simulink model "SUB_CanDm1"  (R2018b)
settings: Solver=VariableStepDiscrete  StartTime=0.0  StopTime=10  RelTol=1e-3
PreLoadFcn:
  | if(exist('MBDS_ModelCallback', 'file'))
  |    MBDS_ModelCallback('PreLoad');
  | end
PostLoadFcn:
  | if(exist('MBDS_ModelCallback', 'file'))
  |    MBDS_ModelCallback('PostLoad');
  | end
InitFcn:
  | if(exist('MBDS_ModelCallback', 'file'))
  |    MBDS_ModelCallback('Init');
  | end
StartFcn:
  | if(exist('MBDS_ModelCallback', 'file'))
  |    MBDS_ModelCallback('Start');
  | end
StopFcn:
  | if(exist('MBDS_ModelCallback', 'file'))
  |    MBDS_ModelCallback('Stop');
  | end
undefined symbols (not defined in the file): sigbuilder_block
libraries: KIBES_Signal x47, simulink x1
(part 2 of 2)

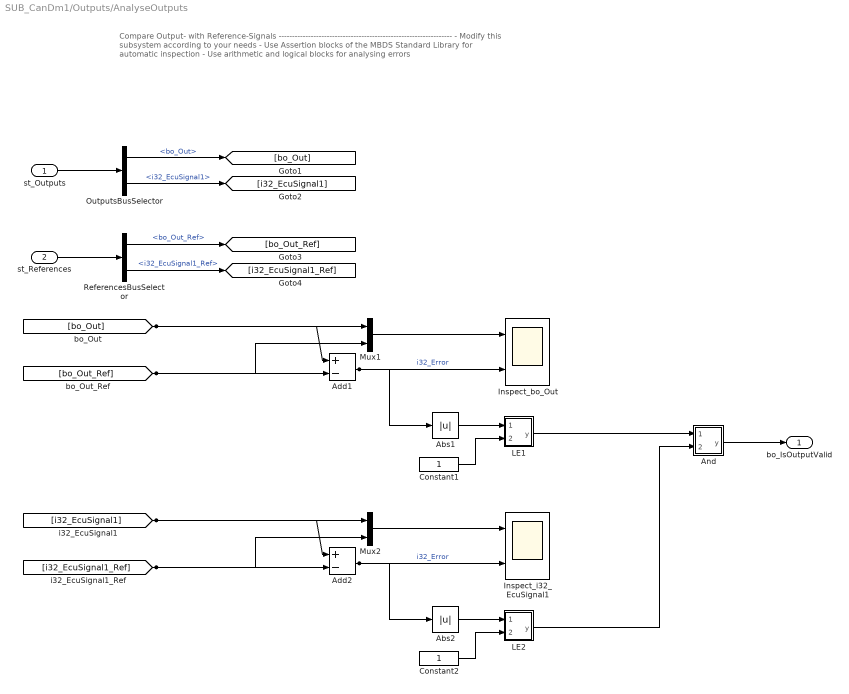
== system SUB_CanDm1/Outputs/AnalyseOutputs ==
  note: Compare Output- with Reference-Signals
      | -----------------------------------------------------------------
      | - Modify this subsystem according to your needs
      | -  Use Assertion blocks of the MBDS Standard Library for automatic inspection
      | - Use arithmetic and logical blocks for analysing errors
  st_Outputs : Inport  InitFcn=|
      | try
      |    MBDS_BlockCallback('Update', gcb);
      | end
  st_References : Inport  InitFcn=|  Port=2
      | try
      |    MBDS_BlockCallback('Update', gcb);
      | end
  Abs1 : Abs  InitFcn=|  OutDataTypeStr=Inherit: Inherit via back propagation
      | if(exist('MBDS_BlockCallback', 'file'))
      |    MBDS_BlockCallback('Update', gcb);  
      | end
      settings: AttributesFormatString=Saturate: %<SaturateOnIntegerOverflow>
  Abs2 : Abs  InitFcn=|  OutDataTypeStr=Inherit: Inherit via back propagation
      | if(exist('MBDS_BlockCallback', 'file'))
      |    MBDS_BlockCallback('Update', gcb);  
      | end
      settings: AttributesFormatString=Saturate: %<SaturateOnIntegerOverflow>
  Add1 : Sum  InitFcn=|  Inputs=+-  OutDataTypeStr=int32  SaturateOnIntegerOverflow=on  InputSameDT=on
      | if(exist('MBDS_BlockCallback', 'file'))
      |    MBDS_BlockCallback('Update', gcb);  
      | end
      settings: AttributesFormatString=Saturate: %<SaturateOnIntegerOverflow>
  Add2 : Sum  InitFcn=|  Inputs=+-  OutDataTypeStr=int32  SaturateOnIntegerOverflow=on  InputSameDT=on
      | if(exist('MBDS_BlockCallback', 'file'))
      |    MBDS_BlockCallback('Update', gcb);  
      | end
      settings: AttributesFormatString=Saturate: %<SaturateOnIntegerOverflow>
  And : Subsystem  InitFcn=|  mask(AND){MBDS_LibraryBlock=on, BitwiseMode=off, Inputs=2, UseBitMask=off, BitMask='A7', OutDataTypeStr=Inherit: Inherit via back propagation, MBDS_BlockVersion=08.20.02}
      | if(exist('MBDS_BlockCallback', 'file'))
      |    MBDS_BlockCallback('Update', gcb);
      | end
      mask prompts: MBDS_LibraryBlock "MBDS library block"; BitwiseMode "Use 'bitwise' mode"; Inputs "Number of input ports:"; UseBitMask "Use bit mask"; BitMask "Bit mask:"; OutDataTypeStr "Output data type:"; MBDS_BlockVersion "Version:"
      mask help: Logical or bitwise AND operator. For multiple inputs, operators are applied across the inputs. For a single input, operators are applied across the input vector. In bitwise mode a bit mask can be applied onto single input signals.
      mask init:
      | if(exist('MBDS_BlockCallback', 'file'))
      |    MBDS_BlockCallback('Init', gcb);
      | else
      |    % Disable all mask parameters
      |    MaskEnables = get_param(gcb, 'MaskEnables');
      |    for k = [1:length(MaskEnables)]
      |       MaskEnables{k} = 'off';
      |    end
      |    if(~isequal(MaskEnables, get_param(gcb, 'MaskEnables')))
      |       set_param(gcb, 'MaskEnables', MaskEnables);
      |    end
      | end
      mask Help: eval(['open([workdir(''library_dir:''),''\Blockset\help\'',get_param(gcb,''MaskType''),''.html''])'])
      mask Callback BitwiseMode:
      | if(exist('MBDS_BlockCallback', 'file'))
      |    MBDS_BlockCallback('BitwiseMode', gcb);
      | end
      mask Callback Inputs:
      | if(exist('MBDS_BlockCallback', 'file'))
      |    MBDS_BlockCallback('Inputs', gcb);
      | end
      mask Callback UseBitMask:
      | if(exist('MBDS_BlockCallback', 'file'))
      |    MBDS_BlockCallback('UseBitMask', gcb);
      | end
      mask Callback BitMask:
      | if(exist('MBDS_BlockCallback', 'file'))
      |    MBDS_BlockCallback('BitMask', gcb);
      | end
      mask TypeOptions OutDataTypeStr: Inherit: Inherit via back propagation | int8 | uint8 | int16 | uint16 | int32 | uint32 | boolean
      mask Callback OutDataTypeStr:
      | % Adopt Value
      | if(exist('MBDS_BlockCallback', 'file'))
      |    MBDS_BlockCallback('OutDataTypeStr', gcb);
      | end
      mask DialogControl ParameterTabVar0 Prompt: Main
      mask DialogControl ParameterTabVar01 Prompt: Signal Attributes
      mask DialogControl ParameterTabVar012 Prompt: Version
      mask Display:
      | % Show icon or block text
      | if(UseBitMask)
      |    if(isnumeric(BitMask))
      |       BitMaskString = ['0x',dec2hex(floor(BitMask))];
      |    elseif(ischar(BitMask))
      |       BitMaskString = ['0x',upper(BitMask)];
      |    else
      |       BitMaskString = '???';
      |    end
      |    disp(sprintf(['AND\n', BitMaskString]))
      | else
      |    disp('AND')
      | end
  Constant1 : Constant  InitFcn=|  OutDataTypeStr=Inherit: Inherit via back propagation
      | if(exist('MBDS_BlockCallback', 'file'))
      |    MBDS_BlockCallback('Update', gcb);  
      | end
  Constant2 : Constant  InitFcn=|  OutDataTypeStr=Inherit: Inherit via back propagation
      | if(exist('MBDS_BlockCallback', 'file'))
      |    MBDS_BlockCallback('Update', gcb);  
      | end
  Inspect_bo_Out : Scope  NumInputPorts=2
  Inspect_i32_EcuSignal1 : Scope  NumInputPorts=2
  LE1 : Subsystem  InitFcn=|  mask(LE){MBDS_LibraryBlock=on, InputSameDT=on, MBDS_BlockVersion=05.20}
      | if(exist('MBDS_BlockCallback', 'file'))
      |    MBDS_BlockCallback('Update', gcb);
      | end
      mask prompts: MBDS_LibraryBlock "MBDS library block"; InputSameDT "Require all inputs to have the same data type"; MBDS_BlockVersion "Block version:"
      mask help: The block compares if the first input signal is lower than or equal to the second input signal.
      mask init: same as SUB_CanDm1/Outputs/AnalyseOutputs/And
      mask Help: eval(['open([workdir(''library_dir:''),''\Blockset\help\'',get_param(gcb,''MaskType''),''.html''])'])
      mask Callback InputSameDT:
      | % Adopt value
      | if(exist('MBDS_BlockCallback', 'file'))
      |    MBDS_BlockCallback('InputSameDT', gcb);
      | end
      mask DialogControl ParameterTabVar0 Prompt: Signal Attributes
      mask DialogControl ParameterTabVar01 Prompt: Version
      mask Display:
      | % Show icon or block text
      | if(exist('MBDS_BlockCallback', 'file'))
      |    image(imread('LE.tif','tif'),[0.33,0.33,0.37,0.37])
      |    disp('')
      | else
      |    disp(sprintf('<='));
      | end
  LE2 : Subsystem  InitFcn=|  mask(LE){MBDS_LibraryBlock=on, InputSameDT=on, MBDS_BlockVersion=05.20}
      | if(exist('MBDS_BlockCallback', 'file'))
      |    MBDS_BlockCallback('Update', gcb);
      | end
      mask prompts: MBDS_LibraryBlock "MBDS library block"; InputSameDT "Require all inputs to have the same data type"; MBDS_BlockVersion "Block version:"
      mask help: The block compares if the first input signal is lower than or equal to the second input signal.
      mask init: same as SUB_CanDm1/Outputs/AnalyseOutputs/And
      mask Help: eval(['open([workdir(''library_dir:''),''\Blockset\help\'',get_param(gcb,''MaskType''),''.html''])'])
      mask Callback InputSameDT:
      | % Adopt value
      | if(exist('MBDS_BlockCallback', 'file'))
      |    MBDS_BlockCallback('InputSameDT', gcb);
      | end
      mask DialogControl ParameterTabVar0 Prompt: Signal Attributes
      mask DialogControl ParameterTabVar01 Prompt: Version
      mask Display:
      | % Show icon or block text
      | if(exist('MBDS_BlockCallback', 'file'))
      |    image(imread('LE.tif','tif'),[0.33,0.33,0.37,0.37])
      |    disp('')
      | else
      |    disp(sprintf('<='));
      | end
  Mux1 : Mux  InitFcn=|  Inputs=2
      | try
      |    MBDS_BlockCallback('Update', gcb);
      | end
  Mux2 : Mux  InitFcn=|  Inputs=2
      | try
      |    MBDS_BlockCallback('Update', gcb);
      | end
  OutputsBusSelector : BusSelector  InitFcn=|  OutputSignals=st_Outputs.bo_Out,i32_EcuSignal1
      | try
      |    MBDS_BlockCallback('Update', gcb);
      | end
  ReferencesBusSelector : BusSelector  InitFcn=|  OutputSignals=st_Outputs.bo_Out_Ref,i32_EcuSignal1_Ref
      | try
      |    MBDS_BlockCallback('Update', gcb);
      | end
  bo_IsOutputValid : Outport  InitFcn=|  PortDimensions=1
      | try
      |    MBDS_BlockCallback('Update', gcb);
      | end
  wires:
  st_Outputs/1 -> OutputsBusSelector/1
  OutputsBusSelector/1 -> [bo_Out]  "<bo_Out>"
  OutputsBusSelector/2 -> [i32_EcuSignal1]  "<i32_EcuSignal1>"
  st_References/1 -> ReferencesBusSelector/1
  ReferencesBusSelector/1 -> [bo_Out_Ref]  "<bo_Out_Ref>"
  ReferencesBusSelector/2 -> [i32_EcuSignal1_Ref]  "<i32_EcuSignal1_Ref>"
  [bo_Out_Ref] -> Add1/2, Mux1/2
  [bo_Out] -> Add1/1, Mux1/1
  Mux1/1 -> Inspect_bo_Out/1
  Add1/1 -> Abs1/1, Inspect_bo_Out/2  "i32_Error"
  Abs1/1 -> LE1/1(u1)
  Constant1/1 -> LE1/2(u2)
  [i32_EcuSignal1_Ref] -> Add2/2, Mux2/2
  [i32_EcuSignal1] -> Add2/1, Mux2/1
  Mux2/1 -> Inspect_i32_EcuSignal1/1
  Add2/1 -> Abs2/1, Inspect_i32_EcuSignal1/2  "i32_Error"
  Abs2/1 -> LE2/1(u1)
  Constant2/1 -> LE2/2(u2)
  And/1(y) -> bo_IsOutputValid/1
  LE1/1(y) -> And/1(u1)
  LE2/1(y) -> And/2(u2)

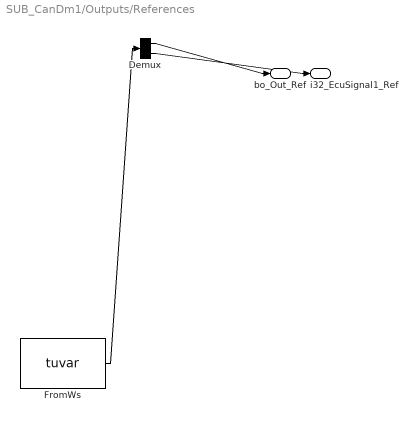
== system SUB_CanDm1/Outputs/References ==
  Demux : Demux  Tag=STV Demux  Outputs=2
  FromWs : FromWorkspace  Tag=STV FromWs  VariableName=tuvar
      SigBuilderData=|
      | dataSet.timeRange = [0 10]
      | dataSet.name = 'TC1'
      | sbobj.Name = 'Signal Builder'
      | sbobj.Groups.Name = 'TC1'
      | sbobj.Groups.Signals(1).Name = 'bo_Out_Ref'
      | sbobj.Groups.Signals(1).XData = [0 1 2 3 4 4 5 6 6 7 8 9 10]
      | sbobj.Groups.Signals(1).YData = [0 0 0 0 0 1 1 1 0 0 0 0 0]
      | sbobj.Groups.Signals(2).Name = 'i32_EcuSignal1_Ref'
      | sbobj.Groups.Signals(2).XData = [0 1 2 3 4 5 6 7 8 9 10]
      | sbobj.Groups.Signals(2).YData = [1 1 1 1 1 1 1 1 1 1 1]
  bo_Out_Ref : Outport  Tag=STV Outport
  i32_EcuSignal1_Ref : Outport  Tag=STV Outport  Port=2
  wires:
  FromWs/1 -> Demux/1
  Demux/1 -> bo_Out_Ref/1
  Demux/2 -> i32_EcuSignal1_Ref/1

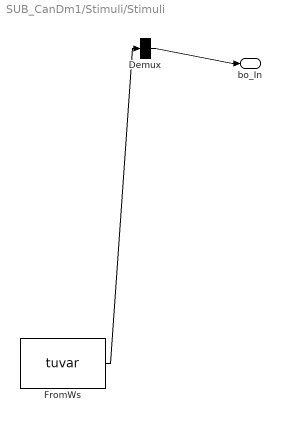
== system SUB_CanDm1/Stimuli/Stimuli ==
  Demux : Demux  Tag=STV Demux  Outputs=1
  FromWs : FromWorkspace  Tag=STV FromWs  VariableName=tuvar
      SigBuilderData=|
      | dataSet.timeRange = [0 10]
      | dataSet.name = 'TC1'
      | sbobj.Name = 'Signal Builder'
      | sbobj.Groups.Name = 'TC1'
      | sbobj.Groups.Signals.Name = 'bo_In'
      | sbobj.Groups.Signals.XData = [0 1 2 3 4 4 5 6 6 7 8 9 10]
      | sbobj.Groups.Signals.YData = [0 0 0 0 0 1 1 1 0 0 0 0 0]
  bo_In : Outport  Tag=STV Outport
  wires:
  FromWs/1 -> Demux/1
  Demux/1 -> bo_In/1

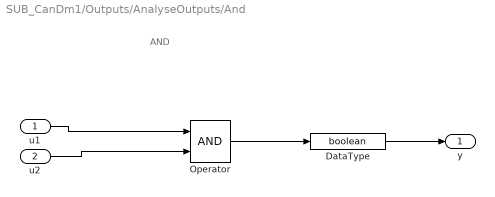
== system SUB_CanDm1/Outputs/AnalyseOutputs/And ==
  note: AND
  u1 : Inport  OutDataTypeStr=boolean
  u2 : Inport  Port=2  OutDataTypeStr=boolean
  DataType : DataTypeConversion  OutDataTypeStr=boolean
  Operator : Logic  AllPortsSameDT=off  OutDataTypeStr=boolean
  y : Outport
  wires:
  Operator/1 -> DataType/1
  u1/1 -> Operator/1
  u2/1 -> Operator/2
  DataType/1 -> y/1

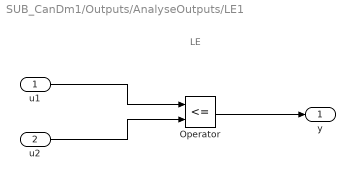
== system SUB_CanDm1/Outputs/AnalyseOutputs/LE1 ==
  note: LE
  u1 : Inport
  u2 : Inport  Port=2
  Operator : RelationalOperator  Operator=<=  OutDataTypeStr=boolean  RndMeth=Nearest  InputSameDT=on
  y : Outport
  wires:
  Operator/1 -> y/1
  u2/1 -> Operator/2
  u1/1 -> Operator/1

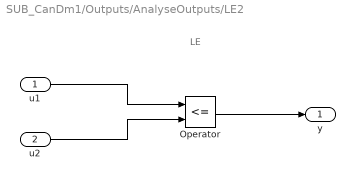
== system SUB_CanDm1/Outputs/AnalyseOutputs/LE2 ==
  note: LE
  u1 : Inport
  u2 : Inport  Port=2
  Operator : RelationalOperator  Operator=<=  OutDataTypeStr=boolean  RndMeth=Nearest  InputSameDT=on
  y : Outport
  wires:
  Operator/1 -> y/1
  u2/1 -> Operator/2
  u1/1 -> Operator/1
